simulink model "Project1part1_abhaykela"  (R2014b)
settings: Solver=ode5  StartTime=0.0  StopTime=tf  FixedStep=0.01  RelTol=1e-3
values from neighbouring files (symbols this model uses):
  x = 2;disp(x)    [HW1.m]    (also in HW2.m = A*cos(w.*t); HW3.m = -5:0.5:5; HW4_1.m = linspace(-2,5); HW4_2a.m = linspace(-2,5))
  xdot = 0    [Project1_AbhayKela_Combined.m]
settings Model: Creator=axk7578  LastModifiedBy=axk7578

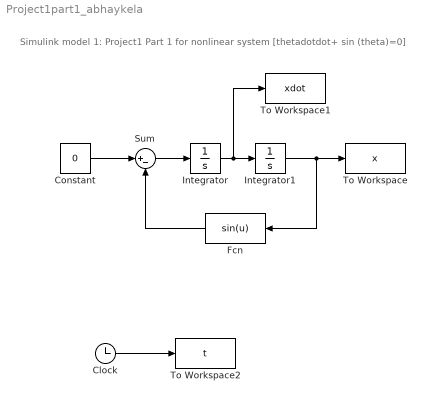
== system Project1part1_abhaykela ==
  note: Simulink model 1: Project1 Part 1 for nonlinear system [thetadotdot+ sin (theta)=0]
  Clock : Clock
  Constant : Constant  Value=0
  Fcn : Fcn  Expr=sin(u)
  Integrator : Integrator  InitialCondition=xdot
  Integrator1 : Integrator  InitialCondition=x
  Sum : Sum  Inputs=|+-
  To Workspace : ToWorkspace  VariableName=x  SampleTime=-1
  To Workspace1 : ToWorkspace  VariableName=xdot  SampleTime=-1
  To Workspace2 : ToWorkspace  VariableName=t  SampleTime=-1
  wires:
  Integrator/1 -> To Workspace1/1, Integrator1/1
  Integrator1/1 -> Fcn/1, To Workspace/1
  Constant/1 -> Sum/1
  Sum/1 -> Integrator/1
  Fcn/1 -> Sum/2
  Clock/1 -> To Workspace2/1
